simulink model "testmdl"  (R2014a)
settings: Solver=ode45  StartTime=0.0  StopTime=10.0  RelTol=1e-3
values from neighbouring files (symbols this model uses):
  gain_act = 1e+2    (= 100)    [demo.m]
  mat1 = [0,-k/m;1,0]    [demo.m]
  mat2 = [k/m,1;0,0]    [demo.m]
  mat3 = [0,1]    [demo.m]
  mat4 = [0,0]    [demo.m]
libraries: cstblocks x1
settings Model: Creator=FYY  LastModifiedBy=FYY

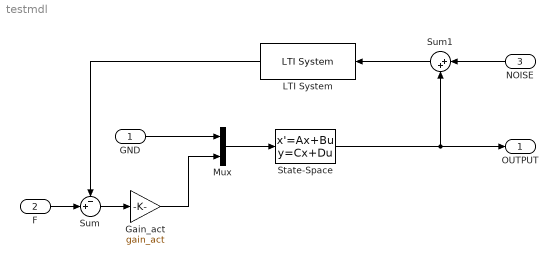
== system testmdl ==
  GND : Inport
  F : Inport  Port=2
  NOISE : Inport  Port=3
  Gain_act : Gain  Gain=gain_act
  LTI System : cstblocks/LTI System  sys=servo  IC=[]
  Mux : Mux  Inputs=2
  State-Space : StateSpace  A=mat1  B=mat2  C=mat3  D=mat4  X0=0
  Sum : Sum  Inputs=-+|
  Sum1 : Sum  Inputs=|++
  OUTPUT : Outport
  wires:
  GND/1 -> Mux/1
  F/1 -> Sum/2
  Mux/1 -> State-Space/1
  State-Space/1 -> Sum1/2, OUTPUT/1
  Gain_act/1 -> Mux/2
  LTI System/1 -> Sum/1
  NOISE/1 -> Sum1/1
  Sum1/1 -> LTI System/1
  Sum/1 -> Gain_act/1
